simulink model "kadai"  (R2019a)
settings: Solver=VariableStepAuto  StartTime=0.0  StopTime=10.0  RelTol=1e-3
undefined symbols (not defined in the file): g, I, L, M, m
settings Model: Creator=robot  LastModifiedBy=robot
settings SolverCC: AlgebraicLoopSolver=LineSearch

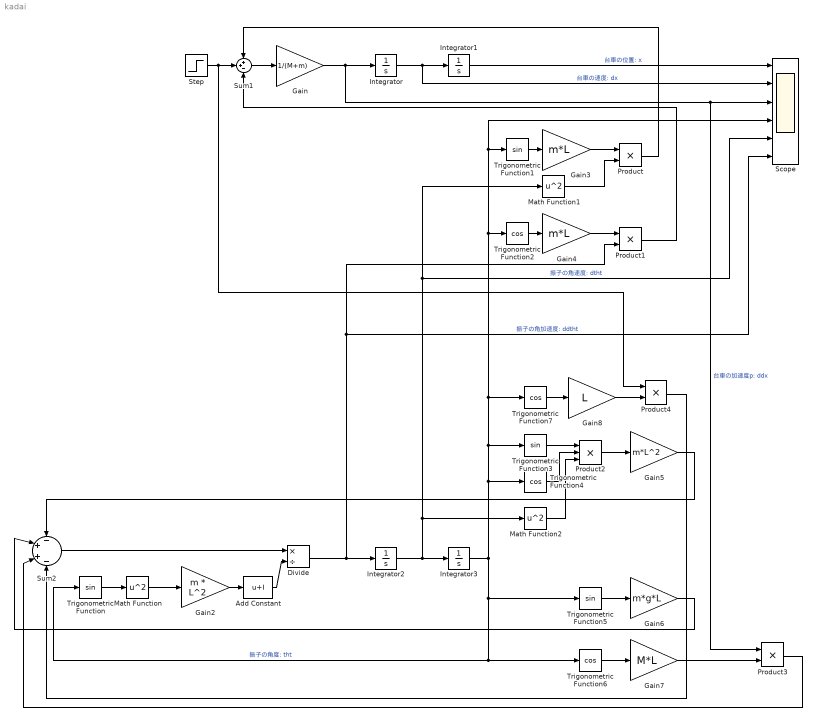
== system kadai ==
  Add Constant : Bias  Bias=I
  Divide : Product  Inputs=*/
  Gain : Gain  Gain=1/(M+m)
  Gain2 : Gain  Gain=m * L^2
  Gain3 : Gain  Gain=m*L
  Gain4 : Gain  Gain=m*L
  Gain5 : Gain  Gain=m*L^2
  Gain6 : Gain  Gain=m*g*L
  Gain7 : Gain  Gain=M*L
  Gain8 : Gain  Gain=L
  Integrator{,1..3} (4 alike) : Integrator
  Math Function : Math  Operator=square  SaturateOnIntegerOverflow=on
  Math Function1 : Math  Operator=square  SaturateOnIntegerOverflow=on
  Math Function2 : Math  Operator=square  SaturateOnIntegerOverflow=on
  Product{,1,3..4} (4 alike) : Product
  Product2 : Product  Inputs=3
  Scope : Scope  NumInputPorts=6
  Step : Step  SampleTime=0
  Sum1 : Sum  Inputs=++-
  Sum2 : Sum  Inputs=-++-
  Trigonometric Function{,1,3,5} (4 alike) : Trigonometry
  Trigonometric Function{2,4,6..7} (4 alike) : Trigonometry  Operator=cos
  wires:
  Gain/1 -> Scope/3, Product3/1, Integrator/1  "台車の加速度p: ddx"
  Integrator/1 -> Scope/2, Integrator1/1  "台車の速度: dx"
  Step/1 -> Product4/1, Sum1/2
  Sum1/1 -> Gain/1
  Trigonometric Function/1 -> Math Function/1
  Divide/1 -> Scope/6, Product1/2, Integrator2/1  "振子の角加速度: ddtht"
  Integrator2/1 -> Math Function2/1, Scope/5, Math Function1/1, Integrator3/1  "振子の角速度: dtht"
  Integrator1/1 -> Scope/1  "台車の位置: x"
  Integrator3/1 -> Trigonometric Function/1, Trigonometric Function6/1, Trigonometric Function5/1, Trigonometric Function4/1, Trigonometric Function3/1, Trigonometric Function7/1, Scope/4, Trigonometric Function1/1, Trigonometric Function2/1  "振子の角度: tht"
  Trigonometric Function1/1 -> Gain3/1
  Math Function1/1 -> Product/2
  Gain3/1 -> Product/1
  Product/1 -> Sum1/1
  Trigonometric Function2/1 -> Gain4/1
  Gain4/1 -> Product1/1
  Product1/1 -> Sum1/3
  Trigonometric Function3/1 -> Product2/1
  Trigonometric Function4/1 -> Product2/2
  Math Function2/1 -> Product2/3
  Product2/1 -> Gain5/1
  Gain5/1 -> Sum2/1
  Trigonometric Function5/1 -> Gain6/1
  Gain6/1 -> Sum2/2
  Trigonometric Function6/1 -> Gain7/1
  Gain7/1 -> Product3/2
  Product3/1 -> Sum2/3
  Trigonometric Function7/1 -> Gain8/1
  Gain8/1 -> Product4/2
  Product4/1 -> Sum2/4
  Sum2/1 -> Divide/1
  Gain2/1 -> Add Constant/1
  Math Function/1 -> Gain2/1
  Add Constant/1 -> Divide/2
